simulink model "gm_Encoder_Zynq_V24"  (R2018a)
settings: Solver=ode3  StartTime=0.0  StopTime=SimulationsDauer  RelTol=1e-3  EnableMultiTasking=on
undefined symbols (not defined in the file or in its folder): DiscIntNeverNeededParam, f_ISR, IncPerTurn, n_max, OmegaPerOverSampl, OverSamplingFactor, OverSamplingFactorInverse, Periode, Phase_Delay_A, Phase_Delay_B, PolePair, QuadratureFactor, T_50MHz, T_mech, TestDrehzahl_rpm
libraries: simulink x2, dspswit3 x2, powerlib_meascontrol x2, simulink_extras x1, powerlib x1
(part 2 of 4)

== system gm_Encoder_Zynq_V24/IncreEncoder_V16/Check_Direction ==
  A : Inport
  B : Inport  Port=2
  Add : Sum  Inputs=+-  AccumDataTypeStr=fixdt(1,4,0)  OutDataTypeStr=fixdt(1,4,0)
  Add1 : Sum  Inputs=+-  AccumDataTypeStr=fixdt(1,4,0)  OutDataTypeStr=fixdt(1,4,0)
  Add2 : Sum  AccumDataTypeStr=fixdt(1,4,0)  OutDataTypeStr=fixdt(1,4,0)
  Change : Sum  AccumDataTypeStr=fixdt(1,4,0)  OutDataTypeStr=fixdt(1,4,0)
  Change1 : Delay  DelayLength=1
  Save_Direction : Switch  Criteria=u2 ~= 0  Threshold=0.1  OutDataTypeStr=Inherit: Inherit via back propagation
  Scope6 : Scope  NumInputPorts=4
  T_count_switch : Switch  Threshold=1  OutDataTypeStr=Inherit: Inherit via back propagation
  TrnLeft : Sum  Inputs=+-  AccumDataTypeStr=fixdt(1,4,0)  OutDataTypeStr=fixdt(1,4,0)
  TrnRight : Sum  Inputs=+-  AccumDataTypeStr=fixdt(1,4,0)  OutDataTypeStr=fixdt(1,4,0)
  TurnLeft : Constant  Value=-1  OutDataTypeStr=fixdt(1,4,0)  SampleTime=-1
  TurnRight : Constant  OutDataTypeStr=fixdt(1,4,0)  SampleTime=-1
  count_old : Delay  DelayLength=1
  count_old1 : Delay  DelayLength=1
  count_old2 : Delay  DelayLength=1
  count_old_switch : Switch  Criteria=u2 ~= 0  OutDataTypeStr=Inherit: Inherit via back propagation
  count_old_switch1 : Switch  Criteria=u2 ~= 0  OutDataTypeStr=Inherit: Inherit via back propagation
  new_value : Delay  DelayLength=1
  nothing : Constant  Value=0  OutDataTypeStr=fixdt(1,4,0)  SampleTime=-1
  nothing1 : Constant  Value=0  OutDataTypeStr=fixdt(1,4,0)  SampleTime=-1
  speed_old_switch : Switch  Threshold=1  OutDataTypeStr=Inherit: Inherit via back propagation
  Dir : Outport
  wires:
  count_old2/1 -> Dir/1, Save_Direction/3
  Change1/1 -> Save_Direction/2, Scope6/3
  Change/1 -> Change1/1
  Add2/1 -> new_value/1, Scope6/4
  speed_old_switch/1 -> Add2/2, Change/2
  nothing1/1 -> T_count_switch/3
  nothing/1 -> speed_old_switch/3
  TurnLeft/1 -> speed_old_switch/1
  TrnLeft/1 -> Scope6/2, speed_old_switch/2
  new_value/1 -> Save_Direction/1
  TrnRight/1 -> T_count_switch/2, Scope6/1
  Add1/1 -> count_old_switch1/2, TrnLeft/1
  count_old1/1 -> Add1/2, count_old_switch1/3
  count_old_switch1/1 -> count_old1/1
  B/1 -> count_old_switch1/1, Add1/1, TrnRight/2
  Save_Direction/1 -> count_old2/1
  T_count_switch/1 -> Add2/1, Change/1
  Add/1 -> count_old_switch/2, TrnRight/1
  TurnRight/1 -> T_count_switch/1
  count_old/1 -> Add/2, count_old_switch/3
  count_old_switch/1 -> count_old/1
  A/1 -> count_old_switch/1, Add/1, TrnLeft/2

== system gm_Encoder_Zynq_V24/IncreEncoder_V16/Counter_speed ==
  note: Count
  note: Reset
  note: Check if count is to big
  note: Check if count is to small
  note: 1 for one cycle if edge recognized
  Enable_ctr : Inport
  Reset : Inport  Port=2
  IncsPerTurn : Inport  Port=3
  Add1 : Sum  AccumDataTypeStr=int16  OutDataTypeStr=uint16
  Constant1 : Constant  Value=0  OutDataTypeStr=uint16  SampleTime=-1
  Constant2 : Constant  OutDataTypeStr=int8  SampleTime=-1
  Constant3 : Constant  Value=0  OutDataTypeStr=int8  SampleTime=-1
  Constant4 : Constant  Value=10  OutDataTypeStr=uint16  SampleTime=-1
  Detec_edge : Sum  Inputs=+-  AccumDataTypeStr=int8  OutDataTypeStr=int8
  Relational Operator : RelationalOperator  OutDataTypeStr=boolean  RndMeth=Nearest
  Reset_flag : Sum  Inputs=+-  AccumDataTypeStr=uint8  OutDataTypeStr=uint8
  Reset_when_overflow : Sum
  Resett_switch1 : Switch  Criteria=u2 ~= 0
  Resett_switch2 : Switch  Criteria=u2 ~= 0
  reset_old{,1..3} (4 alike) : Delay  DelayLength=1
  reset_old_switch : Switch  Criteria=u2 ~= 0
  reset_old_switch1 : Switch  Criteria=u2 ~= 0
  speed_old_switch1 : Switch  Threshold=1
  count : Outport
  wires:
  reset_old3/1 -> Relational Operator/2
  Resett_switch2/1 -> Resett_switch1/3
  IncsPerTurn/1 -> Reset_when_overflow/2
  Constant1/1 -> Resett_switch1/1, Resett_switch2/1
  Relational Operator/1 -> Resett_switch1/2
  Resett_switch1/1 -> reset_old2/1
  Reset_when_overflow/1 -> reset_old3/1
  Constant4/1 -> Reset_when_overflow/1
  Constant2/1 -> speed_old_switch1/1
  Constant3/1 -> speed_old_switch1/3
  speed_old_switch1/1 -> Add1/1
  reset_old2/1 -> count/1, Add1/2, Relational Operator/1
  Add1/1 -> Resett_switch2/3
  Detec_edge/1 -> reset_old_switch1/2, speed_old_switch1/2  "1 for one cycle if edge recognized"
  reset_old1/1 -> Detec_edge/2, reset_old_switch1/3
  reset_old_switch1/1 -> reset_old1/1
  Enable_ctr/1 -> reset_old_switch1/1, Detec_edge/1
  Reset_flag/1 -> Resett_switch2/2, reset_old_switch/2
  reset_old/1 -> Reset_flag/2, reset_old_switch/3
  reset_old_switch/1 -> reset_old/1
  Reset/1 -> reset_old_switch/1, Reset_flag/1

== system gm_Encoder_Zynq_V24/IncreEncoder_V16/Counter_theta ==
  note: Check if count is to small
  note: Check if count is to big
  note: Count
  note: Reset
  note: 1 for one cycle if edge recognized
  Enable_ctr : Inport
  Reset : Inport  Port=2
  IncsPerTurn : Inport  Port=3
  Dir : Inport  Port=4
  Add1 : Sum  AccumDataTypeStr=int16  OutDataTypeStr=int16
  Constant1 : Constant  Value=0  OutDataTypeStr=int16  SampleTime=-1
  Constant2 : Constant  OutDataTypeStr=int16  SampleTime=-1
  Constant3 : Constant  Value=0  OutDataTypeStr=int16  SampleTime=-1
  Constant4 : Constant  Value=10  OutDataTypeStr=int16  SampleTime=-1
  Constant5 : Constant  Value=-1  OutDataTypeStr=int16  SampleTime=-1
  Detec_edge : Sum  Inputs=+-  AccumDataTypeStr=int8  OutDataTypeStr=int8
  Relational Operator : RelationalOperator  Operator=>  OutDataTypeStr=boolean  RndMeth=Nearest
  Relational Operator1 : RelationalOperator  Operator=<=  OutDataTypeStr=boolean  RndMeth=Nearest
  Reset_flag : Sum  Inputs=+-  AccumDataTypeStr=uint8  OutDataTypeStr=uint8
  Reset_when_overflow : Sum  OutDataTypeStr=int16
  Resett_switch1 : Switch  Criteria=u2 ~= 0  OutDataTypeStr=int16
  Resett_switch2 : Switch  Criteria=u2 ~= 0  OutDataTypeStr=int16
  Resett_switch3 : Switch  Criteria=u2 ~= 0  OutDataTypeStr=int16
  only_use_for_neg_speed : Switch  Threshold=1
  reset_old{,1..6} (7 alike) : Delay  DelayLength=1
  reset_old_switch : Switch  Criteria=u2 ~= 0
  reset_old_switch1 : Switch  Criteria=u2 ~= 0
  speed_old_switch1 : Switch  Criteria=u2 ~= 0
  speed_old_switch2 : Switch  Threshold=1
  count : Outport
  wires:
  reset_old6/1 -> speed_old_switch2/2, only_use_for_neg_speed/2
  reset_old5/1 -> Relational Operator/2
  reset_old4/1 -> speed_old_switch1/1
  only_use_for_neg_speed/1 -> Resett_switch3/2
  Relational Operator1/1 -> only_use_for_neg_speed/3
  reset_old2/1 -> Relational Operator1/1
  Resett_switch2/1 -> Resett_switch3/3
  Resett_switch3/1 -> Resett_switch1/3, reset_old2/1
  Constant1/1 -> Relational Operator1/2, only_use_for_neg_speed/1, Resett_switch1/1, Resett_switch2/1
  Relational Operator/1 -> Resett_switch1/2
  Resett_switch1/1 -> reset_old3/1
  reset_old3/1 -> Relational Operator/1, count/1, Add1/2
  speed_old_switch2/1 -> reset_old4/1
  Constant5/1 -> speed_old_switch2/3
  Dir/1 -> reset_old6/1
  IncsPerTurn/1 -> Reset_when_overflow/2, Resett_switch3/1
  Reset_when_overflow/1 -> reset_old5/1
  Constant4/1 -> Reset_when_overflow/1
  Constant2/1 -> speed_old_switch2/1
  Constant3/1 -> speed_old_switch1/3
  speed_old_switch1/1 -> Add1/1
  Add1/1 -> Resett_switch2/3
  Detec_edge/1 -> reset_old_switch1/2, speed_old_switch1/2  "1 for one cycle if edge recognized"
  reset_old1/1 -> Detec_edge/2, reset_old_switch1/3
  reset_old_switch1/1 -> reset_old1/1
  Enable_ctr/1 -> reset_old_switch1/1, Detec_edge/1
  Reset_flag/1 -> Resett_switch2/2, reset_old_switch/2
  reset_old/1 -> Reset_flag/2, reset_old_switch/3
  reset_old_switch/1 -> reset_old/1
  Reset/1 -> reset_old_switch/1, Reset_flag/1

== system gm_Encoder_Zynq_V24/IncreEncoder_V16/Counter_theta_ele ==
  note: Check if count is to small
  note: Check if count is to big
  note: Count
  note: Reset
  note: 1 for one cycle if edge recognized
  Enable_ctr : Inport
  Reset : Inport  Port=2
  IncsPerTurn : Inport  Port=3
  Dir : Inport  Port=4
  Add1 : Sum  AccumDataTypeStr=int16  OutDataTypeStr=int16
  Constant1 : Constant  Value=0  OutDataTypeStr=int16  SampleTime=-1
  Constant2 : Constant  OutDataTypeStr=int16  SampleTime=-1
  Constant3 : Constant  Value=0  OutDataTypeStr=int16  SampleTime=-1
  Constant5 : Constant  Value=-1  OutDataTypeStr=int16  SampleTime=-1
  Detec_edge : Sum  Inputs=+-  AccumDataTypeStr=int8  OutDataTypeStr=int8
  Relational Operator : RelationalOperator  Operator=>  OutDataTypeStr=boolean  RndMeth=Nearest
  Relational Operator1 : RelationalOperator  Operator=<=  OutDataTypeStr=boolean  RndMeth=Nearest
  Reset_flag : Sum  Inputs=+-  AccumDataTypeStr=uint8  OutDataTypeStr=uint8
  Resett_switch1 : Switch  Criteria=u2 ~= 0  OutDataTypeStr=int16
  Resett_switch2 : Switch  Criteria=u2 ~= 0  OutDataTypeStr=int16
  Resett_switch3 : Switch  Criteria=u2 ~= 0  OutDataTypeStr=int16
  only_use_for_neg_speed : Switch  Threshold=1
  reset_old{,1..5} (6 alike) : Delay  DelayLength=1
  reset_old_switch : Switch  Criteria=u2 ~= 0
  reset_old_switch1 : Switch  Criteria=u2 ~= 0
  speed_old_switch1 : Switch  Criteria=u2 ~= 0
  speed_old_switch2 : Switch  Threshold=1
  count : Outport
  wires:
  reset_old5/1 -> only_use_for_neg_speed/2, speed_old_switch2/2
  reset_old4/1 -> speed_old_switch1/1
  only_use_for_neg_speed/1 -> Resett_switch3/2
  Relational Operator1/1 -> only_use_for_neg_speed/3
  reset_old2/1 -> Relational Operator1/1
  Resett_switch2/1 -> Resett_switch3/3
  Resett_switch3/1 -> Resett_switch1/3, reset_old2/1
  Constant1/1 -> Resett_switch1/1, Relational Operator1/2, only_use_for_neg_speed/1, Resett_switch2/1
  Relational Operator/1 -> Resett_switch1/2
  Resett_switch1/1 -> reset_old3/1
  reset_old3/1 -> Relational Operator/1, count/1, Add1/2
  speed_old_switch2/1 -> reset_old4/1
  Constant5/1 -> speed_old_switch2/3
  Dir/1 -> reset_old5/1
  IncsPerTurn/1 -> Relational Operator/2, Resett_switch3/1
  Constant2/1 -> speed_old_switch2/1
  Constant3/1 -> speed_old_switch1/3
  speed_old_switch1/1 -> Add1/1
  Add1/1 -> Resett_switch2/3
  Detec_edge/1 -> reset_old_switch1/2, speed_old_switch1/2  "1 for one cycle if edge recognized"
  reset_old1/1 -> Detec_edge/2, reset_old_switch1/3
  reset_old_switch1/1 -> reset_old1/1
  Enable_ctr/1 -> reset_old_switch1/1, Detec_edge/1
  Reset_flag/1 -> Resett_switch2/2, reset_old_switch/2
  reset_old/1 -> Reset_flag/2, reset_old_switch/3
  reset_old_switch/1 -> reset_old/1
  Reset/1 -> reset_old_switch/1, Reset_flag/1

== system gm_Encoder_Zynq_V24/IncreEncoder_V16/n_aus_theta ==
  count : Inport
  IncsPerTurn : Inport  Port=2
  T : Inport  Port=3
  Add : Sum  Inputs=+-
  Add1 : Sum
  Constant : Constant  Value=0  OutDataTypeStr=fixdt(0,30,24)  SampleTime=-1
  Constant1 : Constant  Value=0  OutDataTypeStr=fixdt(0,30,24)  SampleTime=-1
  Constant2 : Constant  Value=0  OutDataTypeStr=fixdt(0,30,24)  SampleTime=-1
  Gain : Gain  Gain=0.001  ParamDataTypeStr=fixdt(0,16)  OutMin=0  OutMax=0.001*2^16  OutDataTypeStr=fixdt(0,18)
  Product : Product  OutDataTypeStr=Inherit: Same as first input
  ProtectOverflow_T_count : Switch  Threshold=50
  ProtectOverflow_rps : Switch  Threshold=50  OutDataTypeStr=fixdt(0,30,24)
  T_count : Delay  DelayLength=1
  T_count_switch : Switch  Criteria=u2 ~= 0
  count_old : Delay  DelayLength=1
  count_old_switch : Switch  Criteria=u2 ~= 0
  speed_old : Delay  DelayLength=1
  speed_old_switch : Switch  Criteria=u2 ~= 0
  rps : Outport
  wires:
  T_count_switch/1 -> ProtectOverflow_T_count/3, ProtectOverflow_T_count/2, ProtectOverflow_rps/2
  count/1 -> count_old_switch/1, Add/1
  Add1/1 -> T_count_switch/3, Product/1
  Product/1 -> speed_old_switch/1
  T_count/1 -> Add1/2
  ProtectOverflow_T_count/1 -> T_count/1
  T/1 -> Add1/1
  Gain/1 -> Product/2
  IncsPerTurn/1 -> Gain/1
  speed_old/1 -> speed_old_switch/3
  speed_old_switch/1 -> speed_old/1, ProtectOverflow_rps/3
  Constant2/1 -> ProtectOverflow_rps/1
  ProtectOverflow_rps/1 -> rps/1
  Constant1/1 -> ProtectOverflow_T_count/1
  Add/1 -> T_count_switch/2, count_old_switch/2, speed_old_switch/2
  Constant/1 -> T_count_switch/1
  count_old/1 -> Add/2, count_old_switch/3
  count_old_switch/1 -> count_old/1

== system gm_Encoder_Zynq_V24/IncreEncoder_V18/Check_Direction ==
  A : Inport
  B : Inport  Port=2
  Add : Sum  Inputs=+-  AccumDataTypeStr=fixdt(1,4,0)  OutDataTypeStr=fixdt(1,4,0)
  Add1 : Sum  Inputs=+-  AccumDataTypeStr=fixdt(1,4,0)  OutDataTypeStr=fixdt(1,4,0)
  Add2 : Sum  AccumDataTypeStr=fixdt(1,4,0)  OutDataTypeStr=fixdt(1,4,0)
  Change : Sum  AccumDataTypeStr=fixdt(1,4,0)  OutDataTypeStr=fixdt(1,4,0)
  Change1 : Delay  DelayLength=1
  Save_Direction : Switch  Criteria=u2 ~= 0  Threshold=0.1  OutDataTypeStr=Inherit: Inherit via back propagation
  Scope6 : Scope  NumInputPorts=4
  T_count_switch : Switch  Threshold=1  OutDataTypeStr=Inherit: Inherit via back propagation
  TrnLeft : Sum  Inputs=+-  AccumDataTypeStr=fixdt(1,4,0)  OutDataTypeStr=fixdt(1,4,0)
  TrnRight : Sum  Inputs=+-  AccumDataTypeStr=fixdt(1,4,0)  OutDataTypeStr=fixdt(1,4,0)
  TurnLeft : Constant  Value=-1  OutDataTypeStr=fixdt(1,4,0)  SampleTime=-1
  TurnRight : Constant  OutDataTypeStr=fixdt(1,4,0)  SampleTime=-1
  count_old : Delay  DelayLength=1
  count_old1 : Delay  DelayLength=1
  count_old2 : Delay  DelayLength=1
  count_old_switch : Switch  Criteria=u2 ~= 0  OutDataTypeStr=Inherit: Inherit via back propagation
  count_old_switch1 : Switch  Criteria=u2 ~= 0  OutDataTypeStr=Inherit: Inherit via back propagation
  new_value : Delay  DelayLength=1
  nothing : Constant  Value=0  OutDataTypeStr=fixdt(1,4,0)  SampleTime=-1
  nothing1 : Constant  Value=0  OutDataTypeStr=fixdt(1,4,0)  SampleTime=-1
  speed_old_switch : Switch  Threshold=1  OutDataTypeStr=Inherit: Inherit via back propagation
  Dir : Outport
  wires:
  count_old2/1 -> Dir/1, Save_Direction/3
  Change1/1 -> Save_Direction/2, Scope6/3
  Change/1 -> Change1/1
  Add2/1 -> new_value/1, Scope6/4
  speed_old_switch/1 -> Add2/2, Change/2
  nothing1/1 -> T_count_switch/3
  nothing/1 -> speed_old_switch/3
  TurnLeft/1 -> speed_old_switch/1
  TrnLeft/1 -> Scope6/2, speed_old_switch/2
  new_value/1 -> Save_Direction/1
  TrnRight/1 -> T_count_switch/2, Scope6/1
  Add1/1 -> count_old_switch1/2, TrnLeft/1
  count_old1/1 -> Add1/2, count_old_switch1/3
  count_old_switch1/1 -> count_old1/1
  B/1 -> count_old_switch1/1, Add1/1, TrnRight/2
  Save_Direction/1 -> count_old2/1
  T_count_switch/1 -> Add2/1, Change/1
  Add/1 -> count_old_switch/2, TrnRight/1
  TurnRight/1 -> T_count_switch/1
  count_old/1 -> Add/2, count_old_switch/3
  count_old_switch/1 -> count_old/1
  A/1 -> count_old_switch/1, Add/1, TrnLeft/2

== system gm_Encoder_Zynq_V24/IncreEncoder_V18/Counter_speed ==
  note: Count
  note: Reset
  note: Check if count is to big
  note: Check if count is to small
  note: 1 for one cycle if edge recognized
  Enable_ctr : Inport
  Reset : Inport  Port=2
  IncsPerTurn : Inport  Port=3
  Add1 : Sum  AccumDataTypeStr=int16  OutDataTypeStr=uint16
  Constant1 : Constant  Value=0  OutDataTypeStr=uint16  SampleTime=-1
  Constant2 : Constant  OutDataTypeStr=int8  SampleTime=-1
  Constant3 : Constant  Value=0  OutDataTypeStr=int8  SampleTime=-1
  Constant4 : Constant  Value=10  OutDataTypeStr=uint16  SampleTime=-1
  Detec_edge : Sum  Inputs=+-  AccumDataTypeStr=int8  OutDataTypeStr=int8
  Relational Operator : RelationalOperator  OutDataTypeStr=boolean  RndMeth=Nearest
  Reset_flag : Sum  Inputs=+-  AccumDataTypeStr=uint8  OutDataTypeStr=uint8
  Reset_when_overflow : Sum
  Resett_switch1 : Switch  Criteria=u2 ~= 0
  Resett_switch2 : Switch  Criteria=u2 ~= 0
  reset_old{,1..3} (4 alike) : Delay  DelayLength=1
  reset_old_switch : Switch  Criteria=u2 ~= 0
  reset_old_switch1 : Switch  Criteria=u2 ~= 0
  speed_old_switch1 : Switch  Threshold=1
  count : Outport
  wires:
  reset_old3/1 -> Relational Operator/2
  Resett_switch2/1 -> Resett_switch1/3
  IncsPerTurn/1 -> Reset_when_overflow/2
  Constant1/1 -> Resett_switch1/1, Resett_switch2/1
  Relational Operator/1 -> Resett_switch1/2
  Resett_switch1/1 -> reset_old2/1
  Reset_when_overflow/1 -> reset_old3/1
  Constant4/1 -> Reset_when_overflow/1
  Constant2/1 -> speed_old_switch1/1
  Constant3/1 -> speed_old_switch1/3
  speed_old_switch1/1 -> Add1/1
  reset_old2/1 -> count/1, Add1/2, Relational Operator/1
  Add1/1 -> Resett_switch2/3
  Detec_edge/1 -> reset_old_switch1/2, speed_old_switch1/2  "1 for one cycle if edge recognized"
  reset_old1/1 -> Detec_edge/2, reset_old_switch1/3
  reset_old_switch1/1 -> reset_old1/1
  Enable_ctr/1 -> reset_old_switch1/1, Detec_edge/1
  Reset_flag/1 -> Resett_switch2/2, reset_old_switch/2
  reset_old/1 -> Reset_flag/2, reset_old_switch/3
  reset_old_switch/1 -> reset_old/1
  Reset/1 -> reset_old_switch/1, Reset_flag/1

== system gm_Encoder_Zynq_V24/IncreEncoder_V18/Counter_theta ==
  note: Check if count is to small
  note: Check if count is to big
  note: Count
  note: Reset
  note: 1 for one cycle if edge recognized
  Enable_ctr : Inport
  Reset : Inport  Port=2
  IncsPerTurn : Inport  Port=3
  Dir : Inport  Port=4
  Add1 : Sum  AccumDataTypeStr=int16  OutDataTypeStr=int16
  Constant1 : Constant  Value=0  OutDataTypeStr=int16  SampleTime=-1
  Constant2 : Constant  OutDataTypeStr=int16  SampleTime=-1
  Constant3 : Constant  Value=0  OutDataTypeStr=int16  SampleTime=-1
  Constant4 : Constant  Value=10  OutDataTypeStr=int16  SampleTime=-1
  Constant5 : Constant  Value=-1  OutDataTypeStr=int16  SampleTime=-1
  Detec_edge : Sum  Inputs=+-  AccumDataTypeStr=int8  OutDataTypeStr=int8
  Relational Operator : RelationalOperator  Operator=>  OutDataTypeStr=boolean  RndMeth=Nearest
  Relational Operator1 : RelationalOperator  Operator=<=  OutDataTypeStr=boolean  RndMeth=Nearest
  Reset_flag : Sum  Inputs=+-  AccumDataTypeStr=uint8  OutDataTypeStr=uint8
  Reset_when_overflow : Sum  OutDataTypeStr=int16
  Resett_switch1 : Switch  Criteria=u2 ~= 0  OutDataTypeStr=int16
  Resett_switch2 : Switch  Criteria=u2 ~= 0  OutDataTypeStr=int16
  Resett_switch3 : Switch  Criteria=u2 ~= 0  OutDataTypeStr=int16
  only_use_for_neg_speed : Switch  Threshold=1
  reset_old{,1..6} (7 alike) : Delay  DelayLength=1
  reset_old_switch : Switch  Criteria=u2 ~= 0
  reset_old_switch1 : Switch  Criteria=u2 ~= 0
  speed_old_switch1 : Switch  Criteria=u2 ~= 0
  speed_old_switch2 : Switch  Threshold=1
  count : Outport
  wires:
  reset_old6/1 -> speed_old_switch2/2, only_use_for_neg_speed/2
  reset_old5/1 -> Relational Operator/2
  reset_old4/1 -> speed_old_switch1/1
  only_use_for_neg_speed/1 -> Resett_switch3/2
  Relational Operator1/1 -> only_use_for_neg_speed/3
  reset_old2/1 -> Relational Operator1/1
  Resett_switch2/1 -> Resett_switch3/3
  Resett_switch3/1 -> Resett_switch1/3, reset_old2/1
  Constant1/1 -> Relational Operator1/2, only_use_for_neg_speed/1, Resett_switch1/1, Resett_switch2/1
  Relational Operator/1 -> Resett_switch1/2
  Resett_switch1/1 -> reset_old3/1
  reset_old3/1 -> Relational Operator/1, count/1, Add1/2
  speed_old_switch2/1 -> reset_old4/1
  Constant5/1 -> speed_old_switch2/3
  Dir/1 -> reset_old6/1
  IncsPerTurn/1 -> Reset_when_overflow/2, Resett_switch3/1
  Reset_when_overflow/1 -> reset_old5/1
  Constant4/1 -> Reset_when_overflow/1
  Constant2/1 -> speed_old_switch2/1
  Constant3/1 -> speed_old_switch1/3
  speed_old_switch1/1 -> Add1/1
  Add1/1 -> Resett_switch2/3
  Detec_edge/1 -> reset_old_switch1/2, speed_old_switch1/2  "1 for one cycle if edge recognized"
  reset_old1/1 -> Detec_edge/2, reset_old_switch1/3
  reset_old_switch1/1 -> reset_old1/1
  Enable_ctr/1 -> reset_old_switch1/1, Detec_edge/1
  Reset_flag/1 -> Resett_switch2/2, reset_old_switch/2
  reset_old/1 -> Reset_flag/2, reset_old_switch/3
  reset_old_switch/1 -> reset_old/1
  Reset/1 -> reset_old_switch/1, Reset_flag/1

== system gm_Encoder_Zynq_V24/IncreEncoder_V18/Counter_theta_ele ==
  note: Check if count is to small
  note: Check if count is to big
  note: Count
  note: Reset
  note: 1 for one cycle if edge recognized
  Enable_ctr : Inport
  Reset : Inport  Port=2
  IncsPerTurn : Inport  Port=3
  Dir : Inport  Port=4
  Add1 : Sum  AccumDataTypeStr=int16  OutDataTypeStr=int16
  Constant1 : Constant  Value=0  OutDataTypeStr=int16  SampleTime=-1
  Constant2 : Constant  OutDataTypeStr=int16  SampleTime=-1
  Constant3 : Constant  Value=0  OutDataTypeStr=int16  SampleTime=-1
  Constant5 : Constant  Value=-1  OutDataTypeStr=int16  SampleTime=-1
  Detec_edge : Sum  Inputs=+-  AccumDataTypeStr=int8  OutDataTypeStr=int8
  Relational Operator : RelationalOperator  Operator=>  OutDataTypeStr=boolean  RndMeth=Nearest
  Relational Operator1 : RelationalOperator  Operator=<=  OutDataTypeStr=boolean  RndMeth=Nearest
  Reset_flag : Sum  Inputs=+-  AccumDataTypeStr=uint8  OutDataTypeStr=uint8
  Resett_switch1 : Switch  Criteria=u2 ~= 0  OutDataTypeStr=int16
  Resett_switch2 : Switch  Criteria=u2 ~= 0  OutDataTypeStr=int16
  Resett_switch3 : Switch  Criteria=u2 ~= 0  OutDataTypeStr=int16
  only_use_for_neg_speed : Switch  Threshold=1
  reset_old{,1..5} (6 alike) : Delay  DelayLength=1
  reset_old_switch : Switch  Criteria=u2 ~= 0
  reset_old_switch1 : Switch  Criteria=u2 ~= 0
  speed_old_switch1 : Switch  Criteria=u2 ~= 0
  speed_old_switch2 : Switch  Threshold=1
  count : Outport
  wires:
  reset_old5/1 -> only_use_for_neg_speed/2, speed_old_switch2/2
  reset_old4/1 -> speed_old_switch1/1
  only_use_for_neg_speed/1 -> Resett_switch3/2
  Relational Operator1/1 -> only_use_for_neg_speed/3
  reset_old2/1 -> Relational Operator1/1
  Resett_switch2/1 -> Resett_switch3/3
  Resett_switch3/1 -> Resett_switch1/3, reset_old2/1
  Constant1/1 -> Resett_switch1/1, Relational Operator1/2, only_use_for_neg_speed/1, Resett_switch2/1
  Relational Operator/1 -> Resett_switch1/2
  Resett_switch1/1 -> reset_old3/1
  reset_old3/1 -> Relational Operator/1, count/1, Add1/2
  speed_old_switch2/1 -> reset_old4/1
  Constant5/1 -> speed_old_switch2/3
  Dir/1 -> reset_old5/1
  IncsPerTurn/1 -> Relational Operator/2, Resett_switch3/1
  Constant2/1 -> speed_old_switch2/1
  Constant3/1 -> speed_old_switch1/3
  speed_old_switch1/1 -> Add1/1
  Add1/1 -> Resett_switch2/3
  Detec_edge/1 -> reset_old_switch1/2, speed_old_switch1/2  "1 for one cycle if edge recognized"
  reset_old1/1 -> Detec_edge/2, reset_old_switch1/3
  reset_old_switch1/1 -> reset_old1/1
  Enable_ctr/1 -> reset_old_switch1/1, Detec_edge/1
  Reset_flag/1 -> Resett_switch2/2, reset_old_switch/2
  reset_old/1 -> Reset_flag/2, reset_old_switch/3
  reset_old_switch/1 -> reset_old/1
  Reset/1 -> reset_old_switch/1, Reset_flag/1

== system gm_Encoder_Zynq_V24/IncreEncoder_V18/n_aus_theta ==
  count : Inport
  IncsPerTurn : Inport  Port=2
  T : Inport  Port=3
  Add : Sum  Inputs=+-
  Add1 : Sum
  Constant : Constant  Value=0  OutDataTypeStr=fixdt(0,30,24)  SampleTime=-1
  Constant1 : Constant  Value=0  OutDataTypeStr=fixdt(0,30,24)  SampleTime=-1
  Constant2 : Constant  Value=0  OutDataTypeStr=fixdt(0,30,24)  SampleTime=-1
  Gain : Gain  Gain=0.001  ParamDataTypeStr=fixdt(0,16)  OutMin=0  OutMax=0.001*2^16  OutDataTypeStr=fixdt(0,18)
  Product : Product  OutDataTypeStr=Inherit: Same as first input
  ProtectOverflow_T_count : Switch  Threshold=50
  ProtectOverflow_rps : Switch  Threshold=50  OutDataTypeStr=fixdt(0,30,24)
  T_count : Delay  DelayLength=1
  T_count_switch : Switch  Criteria=u2 ~= 0
  count_old : Delay  DelayLength=1
  count_old_switch : Switch  Criteria=u2 ~= 0
  speed_old : Delay  DelayLength=1
  speed_old_switch : Switch  Criteria=u2 ~= 0
  rps : Outport
  wires:
  T_count_switch/1 -> ProtectOverflow_T_count/3, ProtectOverflow_T_count/2, ProtectOverflow_rps/2
  count/1 -> count_old_switch/1, Add/1
  Add1/1 -> T_count_switch/3, Product/1
  Product/1 -> speed_old_switch/1
  T_count/1 -> Add1/2
  ProtectOverflow_T_count/1 -> T_count/1
  T/1 -> Add1/1
  Gain/1 -> Product/2
  IncsPerTurn/1 -> Gain/1
  speed_old/1 -> speed_old_switch/3
  speed_old_switch/1 -> speed_old/1, ProtectOverflow_rps/3
  Constant2/1 -> ProtectOverflow_rps/1
  ProtectOverflow_rps/1 -> rps/1
  Constant1/1 -> ProtectOverflow_T_count/1
  Add/1 -> T_count_switch/2, count_old_switch/2, speed_old_switch/2
  Constant/1 -> T_count_switch/1
  count_old/1 -> Add/2, count_old_switch/3
  count_old_switch/1 -> count_old/1

== system gm_Encoder_Zynq_V24/IncreEncoder_V19/Check_Direction ==
  A : Inport
  B : Inport  Port=2
  Add : Sum  Inputs=+-  AccumDataTypeStr=fixdt(1,4,0)  OutDataTypeStr=fixdt(1,4,0)
  Add1 : Sum  Inputs=+-  AccumDataTypeStr=fixdt(1,4,0)  OutDataTypeStr=fixdt(1,4,0)
  Add2 : Sum  AccumDataTypeStr=fixdt(1,4,0)  OutDataTypeStr=fixdt(1,4,0)
  Change : Sum  AccumDataTypeStr=fixdt(1,4,0)  OutDataTypeStr=fixdt(1,4,0)
  Change1 : Delay  DelayLength=1
  Save_Direction : Switch  Criteria=u2 ~= 0  Threshold=0.1  OutDataTypeStr=Inherit: Inherit via back propagation
  Scope6 : Scope  NumInputPorts=4
  T_count_switch : Switch  Threshold=1  OutDataTypeStr=Inherit: Inherit via back propagation
  TrnLeft : Sum  Inputs=+-  AccumDataTypeStr=fixdt(1,4,0)  OutDataTypeStr=fixdt(1,4,0)
  TrnRight : Sum  Inputs=+-  AccumDataTypeStr=fixdt(1,4,0)  OutDataTypeStr=fixdt(1,4,0)
  TurnLeft : Constant  Value=-1  OutDataTypeStr=fixdt(1,4,0)  SampleTime=-1
  TurnRight : Constant  OutDataTypeStr=fixdt(1,4,0)  SampleTime=-1
  count_old : Delay  DelayLength=1
  count_old1 : Delay  DelayLength=1
  count_old2 : Delay  DelayLength=1
  count_old_switch : Switch  Criteria=u2 ~= 0  OutDataTypeStr=Inherit: Inherit via back propagation
  count_old_switch1 : Switch  Criteria=u2 ~= 0  OutDataTypeStr=Inherit: Inherit via back propagation
  new_value : Delay  DelayLength=1
  nothing : Constant  Value=0  OutDataTypeStr=fixdt(1,4,0)  SampleTime=-1
  nothing1 : Constant  Value=0  OutDataTypeStr=fixdt(1,4,0)  SampleTime=-1
  speed_old_switch : Switch  Threshold=1  OutDataTypeStr=Inherit: Inherit via back propagation
  Dir : Outport
  wires:
  count_old2/1 -> Dir/1, Save_Direction/3
  Change1/1 -> Save_Direction/2, Scope6/3
  Change/1 -> Change1/1
  Add2/1 -> new_value/1, Scope6/4
  speed_old_switch/1 -> Add2/2, Change/2
  nothing1/1 -> T_count_switch/3
  nothing/1 -> speed_old_switch/3
  TurnLeft/1 -> speed_old_switch/1
  TrnLeft/1 -> Scope6/2, speed_old_switch/2
  new_value/1 -> Save_Direction/1
  TrnRight/1 -> T_count_switch/2, Scope6/1
  Add1/1 -> count_old_switch1/2, TrnLeft/1
  count_old1/1 -> Add1/2, count_old_switch1/3
  count_old_switch1/1 -> count_old1/1
  B/1 -> count_old_switch1/1, Add1/1, TrnRight/2
  Save_Direction/1 -> count_old2/1
  T_count_switch/1 -> Add2/1, Change/1
  Add/1 -> count_old_switch/2, TrnRight/1
  TurnRight/1 -> T_count_switch/1
  count_old/1 -> Add/2, count_old_switch/3
  count_old_switch/1 -> count_old/1
  A/1 -> count_old_switch/1, Add/1, TrnLeft/2

== system gm_Encoder_Zynq_V24/IncreEncoder_V19/Counter_speed ==
  note: Count
  note: Reset
  note: Check if count is to big
  note: Check if count is to small
  note: 1 for one cycle if edge recognized
  Enable_ctr : Inport
  Reset : Inport  Port=2
  IncsPerTurn : Inport  Port=3
  Add1 : Sum  AccumDataTypeStr=int16  OutDataTypeStr=uint16
  Constant1 : Constant  Value=0  OutDataTypeStr=uint16  SampleTime=-1
  Constant2 : Constant  OutDataTypeStr=int8  SampleTime=-1
  Constant3 : Constant  Value=0  OutDataTypeStr=int8  SampleTime=-1
  Constant4 : Constant  Value=10  OutDataTypeStr=uint16  SampleTime=-1
  Detec_edge : Sum  Inputs=+-  AccumDataTypeStr=int8  OutDataTypeStr=int8
  Relational Operator : RelationalOperator  OutDataTypeStr=boolean  RndMeth=Nearest
  Reset_flag : Sum  Inputs=+-  AccumDataTypeStr=uint8  OutDataTypeStr=uint8
  Reset_when_overflow : Sum
  Resett_switch1 : Switch  Criteria=u2 ~= 0
  Resett_switch2 : Switch  Criteria=u2 ~= 0
  reset_old{,1..3} (4 alike) : Delay  DelayLength=1
  reset_old_switch : Switch  Criteria=u2 ~= 0
  reset_old_switch1 : Switch  Criteria=u2 ~= 0
  speed_old_switch1 : Switch  Threshold=1
  count : Outport
  wires:
  reset_old3/1 -> Relational Operator/2
  Resett_switch2/1 -> Resett_switch1/3
  IncsPerTurn/1 -> Reset_when_overflow/2
  Constant1/1 -> Resett_switch1/1, Resett_switch2/1
  Relational Operator/1 -> Resett_switch1/2
  Resett_switch1/1 -> reset_old2/1
  Reset_when_overflow/1 -> reset_old3/1
  Constant4/1 -> Reset_when_overflow/1
  Constant2/1 -> speed_old_switch1/1
  Constant3/1 -> speed_old_switch1/3
  speed_old_switch1/1 -> Add1/1
  reset_old2/1 -> count/1, Add1/2, Relational Operator/1
  Add1/1 -> Resett_switch2/3
  Detec_edge/1 -> reset_old_switch1/2, speed_old_switch1/2  "1 for one cycle if edge recognized"
  reset_old1/1 -> Detec_edge/2, reset_old_switch1/3
  reset_old_switch1/1 -> reset_old1/1
  Enable_ctr/1 -> reset_old_switch1/1, Detec_edge/1
  Reset_flag/1 -> Resett_switch2/2, reset_old_switch/2
  reset_old/1 -> Reset_flag/2, reset_old_switch/3
  reset_old_switch/1 -> reset_old/1
  Reset/1 -> reset_old_switch/1, Reset_flag/1

== system gm_Encoder_Zynq_V24/IncreEncoder_V19/Counter_theta ==
  note: Check if count is to small
  note: Check if count is to big
  note: Count
  note: Reset
  note: 1 for one cycle if edge recognized
  Enable_ctr : Inport
  Reset : Inport  Port=2
  IncsPerTurn : Inport  Port=3
  Dir : Inport  Port=4
  Add1 : Sum  AccumDataTypeStr=int16  OutDataTypeStr=int16
  Constant1 : Constant  Value=0  OutDataTypeStr=int16  SampleTime=-1
  Constant2 : Constant  OutDataTypeStr=int16  SampleTime=-1
  Constant3 : Constant  Value=0  OutDataTypeStr=int16  SampleTime=-1
  Constant4 : Constant  Value=10  OutDataTypeStr=int16  SampleTime=-1
  Constant5 : Constant  Value=-1  OutDataTypeStr=int16  SampleTime=-1
  Detec_edge : Sum  Inputs=+-  AccumDataTypeStr=int8  OutDataTypeStr=int8
  Relational Operator : RelationalOperator  Operator=>  OutDataTypeStr=boolean  RndMeth=Nearest
  Relational Operator1 : RelationalOperator  Operator=<=  OutDataTypeStr=boolean  RndMeth=Nearest
  Reset_flag : Sum  Inputs=+-  AccumDataTypeStr=uint8  OutDataTypeStr=uint8
  Reset_when_overflow : Sum  OutDataTypeStr=int16
  Resett_switch1 : Switch  Criteria=u2 ~= 0  OutDataTypeStr=int16
  Resett_switch2 : Switch  Criteria=u2 ~= 0  OutDataTypeStr=int16
  Resett_switch3 : Switch  Criteria=u2 ~= 0  OutDataTypeStr=int16
  only_use_for_neg_speed : Switch  Threshold=1
  reset_old{,1..6} (7 alike) : Delay  DelayLength=1
  reset_old_switch : Switch  Criteria=u2 ~= 0
  reset_old_switch1 : Switch  Criteria=u2 ~= 0
  speed_old_switch1 : Switch  Criteria=u2 ~= 0
  speed_old_switch2 : Switch  Threshold=1
  count : Outport
  wires:
  reset_old6/1 -> speed_old_switch2/2, only_use_for_neg_speed/2
  reset_old5/1 -> Relational Operator/2
  reset_old4/1 -> speed_old_switch1/1
  only_use_for_neg_speed/1 -> Resett_switch3/2
  Relational Operator1/1 -> only_use_for_neg_speed/3
  reset_old2/1 -> Relational Operator1/1
  Resett_switch2/1 -> Resett_switch3/3
  Resett_switch3/1 -> Resett_switch1/3, reset_old2/1
  Constant1/1 -> Relational Operator1/2, only_use_for_neg_speed/1, Resett_switch1/1, Resett_switch2/1
  Relational Operator/1 -> Resett_switch1/2
  Resett_switch1/1 -> reset_old3/1
  reset_old3/1 -> Relational Operator/1, count/1, Add1/2
  speed_old_switch2/1 -> reset_old4/1
  Constant5/1 -> speed_old_switch2/3
  Dir/1 -> reset_old6/1
  IncsPerTurn/1 -> Reset_when_overflow/2, Resett_switch3/1
  Reset_when_overflow/1 -> reset_old5/1
  Constant4/1 -> Reset_when_overflow/1
  Constant2/1 -> speed_old_switch2/1
  Constant3/1 -> speed_old_switch1/3
  speed_old_switch1/1 -> Add1/1
  Add1/1 -> Resett_switch2/3
  Detec_edge/1 -> reset_old_switch1/2, speed_old_switch1/2  "1 for one cycle if edge recognized"
  reset_old1/1 -> Detec_edge/2, reset_old_switch1/3
  reset_old_switch1/1 -> reset_old1/1
  Enable_ctr/1 -> reset_old_switch1/1, Detec_edge/1
  Reset_flag/1 -> Resett_switch2/2, reset_old_switch/2
  reset_old/1 -> Reset_flag/2, reset_old_switch/3
  reset_old_switch/1 -> reset_old/1
  Reset/1 -> reset_old_switch/1, Reset_flag/1

== system gm_Encoder_Zynq_V24/IncreEncoder_V19/Counter_theta_ele ==
  note: Check if count is to small
  note: Check if count is to big
  note: Count
  note: Reset
  note: 1 for one cycle if edge recognized
  Enable_ctr : Inport
  Reset : Inport  Port=2
  IncsPerTurn : Inport  Port=3
  Dir : Inport  Port=4
  Add1 : Sum  AccumDataTypeStr=int16  OutDataTypeStr=int16
  Constant1 : Constant  Value=0  OutDataTypeStr=int16  SampleTime=-1
  Constant2 : Constant  OutDataTypeStr=int16  SampleTime=-1
  Constant3 : Constant  Value=0  OutDataTypeStr=int16  SampleTime=-1
  Constant5 : Constant  Value=-1  OutDataTypeStr=int16  SampleTime=-1
  Detec_edge : Sum  Inputs=+-  AccumDataTypeStr=int8  OutDataTypeStr=int8
  Relational Operator : RelationalOperator  Operator=>  OutDataTypeStr=boolean  RndMeth=Nearest
  Relational Operator1 : RelationalOperator  Operator=<=  OutDataTypeStr=boolean  RndMeth=Nearest
  Reset_flag : Sum  Inputs=+-  AccumDataTypeStr=uint8  OutDataTypeStr=uint8
  Resett_switch1 : Switch  Criteria=u2 ~= 0  OutDataTypeStr=int16
  Resett_switch2 : Switch  Criteria=u2 ~= 0  OutDataTypeStr=int16
  Resett_switch3 : Switch  Criteria=u2 ~= 0  OutDataTypeStr=int16
  only_use_for_neg_speed : Switch  Threshold=1
  reset_old{,1..5} (6 alike) : Delay  DelayLength=1
  reset_old_switch : Switch  Criteria=u2 ~= 0
  reset_old_switch1 : Switch  Criteria=u2 ~= 0
  speed_old_switch1 : Switch  Criteria=u2 ~= 0
  speed_old_switch2 : Switch  Threshold=1
  count : Outport
  wires:
  reset_old5/1 -> only_use_for_neg_speed/2, speed_old_switch2/2
  reset_old4/1 -> speed_old_switch1/1
  only_use_for_neg_speed/1 -> Resett_switch3/2
  Relational Operator1/1 -> only_use_for_neg_speed/3
  reset_old2/1 -> Relational Operator1/1
  Resett_switch2/1 -> Resett_switch3/3
  Resett_switch3/1 -> Resett_switch1/3, reset_old2/1
  Constant1/1 -> Resett_switch1/1, Relational Operator1/2, only_use_for_neg_speed/1, Resett_switch2/1
  Relational Operator/1 -> Resett_switch1/2
  Resett_switch1/1 -> reset_old3/1
  reset_old3/1 -> Relational Operator/1, count/1, Add1/2
  speed_old_switch2/1 -> reset_old4/1
  Constant5/1 -> speed_old_switch2/3
  Dir/1 -> reset_old5/1
  IncsPerTurn/1 -> Relational Operator/2, Resett_switch3/1
  Constant2/1 -> speed_old_switch2/1
  Constant3/1 -> speed_old_switch1/3
  speed_old_switch1/1 -> Add1/1
  Add1/1 -> Resett_switch2/3
  Detec_edge/1 -> reset_old_switch1/2, speed_old_switch1/2  "1 for one cycle if edge recognized"
  reset_old1/1 -> Detec_edge/2, reset_old_switch1/3
  reset_old_switch1/1 -> reset_old1/1
  Enable_ctr/1 -> reset_old_switch1/1, Detec_edge/1
  Reset_flag/1 -> Resett_switch2/2, reset_old_switch/2
  reset_old/1 -> Reset_flag/2, reset_old_switch/3
  reset_old_switch/1 -> reset_old/1
  Reset/1 -> reset_old_switch/1, Reset_flag/1

== system gm_Encoder_Zynq_V24/IncreEncoder_V19/n_aus_theta ==
  note: Detect each edge of the encoder
  count : Inport
  T : Inport  Port=2
  ProtectThetaLimit : Inport  Port=3
  Add : Sum  Inputs=+-
  Add1 : Sum
  Constant : Constant  Value=0  OutDataTypeStr=fixdt(0,30,24)  SampleTime=-1
  Constant1 : Constant  Value=0  OutDataTypeStr=fixdt(0,30,24)  SampleTime=-1
  Constant2 : Constant  Value=0  OutDataTypeStr=fixdt(0,30,24)  SampleTime=-1
  Logical Operator : Logic  AllPortsSameDT=off  OutDataTypeStr=boolean
  ProtectOverflow_T_count : Switch  Threshold=50
  ProtectOverflow_rps : Switch  Threshold=50  OutDataTypeStr=fixdt(0,30,24)
  ProtectToUseOmegaIfThetaJump : RelationalOperator  OutDataTypeStr=boolean  RndMeth=Nearest
  T_count : Delay  DelayLength=1
  T_count_switch : Switch  Criteria=u2 ~= 0
  count_old : Delay  DelayLength=1
  count_old_switch : Switch  Criteria=u2 ~= 0
  speed_old : Delay  DelayLength=1
  speed_old_switch : Switch  Criteria=u2 ~= 0
  rps : Outport
  wires:
  ProtectThetaLimit/1 -> ProtectToUseOmegaIfThetaJump/2
  Logical Operator/1 -> speed_old_switch/2
  ProtectToUseOmegaIfThetaJump/1 -> Logical Operator/2
  T_count_switch/1 -> ProtectOverflow_T_count/3, ProtectOverflow_T_count/2, ProtectOverflow_rps/2
  count/1 -> count_old_switch/1, Add/1, ProtectToUseOmegaIfThetaJump/1
  Add1/1 -> T_count_switch/3, speed_old_switch/1
  T_count/1 -> Add1/2
  ProtectOverflow_T_count/1 -> T_count/1
  T/1 -> Add1/1
  speed_old/1 -> speed_old_switch/3
  speed_old_switch/1 -> speed_old/1, ProtectOverflow_rps/3
  Constant2/1 -> ProtectOverflow_rps/1
  ProtectOverflow_rps/1 -> rps/1
  Constant1/1 -> ProtectOverflow_T_count/1
  Add/1 -> T_count_switch/2, Logical Operator/1, count_old_switch/2
  Constant/1 -> T_count_switch/1
  count_old/1 -> Add/2, count_old_switch/3
  count_old_switch/1 -> count_old/1

== system gm_Encoder_Zynq_V24/IncreEncoder_V22/Average ==
  note: Maximum of the OverSampling is 6
  "OmegaIn " : Inport
  NewMeasurement : Inport  Port=2
  SamplingFactorInv : Inport  Port=3
  SamplingFactor : Inport  Port=4
  Add : Sum  Inputs=++++++  OutDataTypeStr=Inherit: Same as first input
  Ask1 : Switch  Threshold=fi(2,0,4,0)  OutDataTypeStr=fixdt(1,24,11)
  Ask2 : Switch  Threshold=fi(3,0,4,0)  OutDataTypeStr=fixdt(1,24,11)
  Ask3 : Switch  Threshold=fi(4,0,4,0)  OutDataTypeStr=fixdt(1,24,11)
  Ask4 : Switch  Threshold=fi(5,0,4,0)  OutDataTypeStr=fixdt(1,24,11)
  Ask5 : Switch  Threshold=fi(6,0,4,0)  OutDataTypeStr=fixdt(1,24,11)
  Constant1 : Constant  Value=0  OutDataTypeStr=fixdt(1,24,11)  SampleTime=-1
  NewSpeed{,1..4} (5 alike) : Switch  Criteria=u2 ~= 0  Threshold=0.5  OutDataTypeStr=fixdt(1,24,11)
  Product : Product  OutDataTypeStr=Inherit: Same as first input
  hold{,1..4} (5 alike) : Delay  DelayLength=1
  OmegaOut : Outport
  wires:
  SamplingFactor/1 -> Ask5/2, Ask4/2, Ask3/2, Ask2/2, Ask1/2
  Ask5/1 -> Add/6
  Ask4/1 -> Add/5
  Ask3/1 -> Add/4
  Ask2/1 -> Add/3
  Ask1/1 -> Add/2
  Constant1/1 -> Ask1/3, Ask2/3, Ask3/3, Ask4/3, Ask5/3
  hold4/1 -> NewSpeed4/3
  NewSpeed4/1 -> Ask5/1, hold4/1
  hold3/1 -> NewSpeed3/3, NewSpeed4/1
  NewSpeed3/1 -> Ask4/1, hold3/1
  NewMeasurement/1 -> NewSpeed/2, NewSpeed1/2, NewSpeed2/2, NewSpeed3/2, NewSpeed4/2
  NewSpeed2/1 -> Ask3/1, hold2/1
  hold2/1 -> NewSpeed2/3, NewSpeed3/1
  hold1/1 -> NewSpeed1/3, NewSpeed2/1
  NewSpeed1/1 -> Ask2/1, hold1/1
  NewSpeed/1 -> Ask1/1, hold/1
  hold/1 -> NewSpeed/3, NewSpeed1/1
  Add/1 -> Product/1
  SamplingFactorInv/1 -> Product/2
  "OmegaIn "/1 -> NewSpeed/1, Add/1
  Product/1 -> OmegaOut/1

== system gm_Encoder_Zynq_V24/IncreEncoder_V22/Check_Direction ==
  A : Inport
  B : Inport  Port=2
  Add : Sum  Inputs=+-  AccumDataTypeStr=fixdt(1,4,0)  OutDataTypeStr=fixdt(1,4,0)
  Add1 : Sum  Inputs=+-  AccumDataTypeStr=fixdt(1,4,0)  OutDataTypeStr=fixdt(1,4,0)
  Add2 : Sum  AccumDataTypeStr=fixdt(1,4,0)  OutDataTypeStr=fixdt(1,4,0)
  Change : Sum  AccumDataTypeStr=fixdt(1,4,0)  OutDataTypeStr=fixdt(1,4,0)
  Change1 : Delay  DelayLength=1
  Save_Direction : Switch  Criteria=u2 ~= 0  Threshold=0.1  OutDataTypeStr=Inherit: Inherit via back propagation
  T_count_switch : Switch  Threshold=1  OutDataTypeStr=Inherit: Inherit via back propagation
  TrnLeft : Sum  Inputs=+-  AccumDataTypeStr=fixdt(1,4,0)  OutDataTypeStr=fixdt(1,4,0)
  TrnRight : Sum  Inputs=+-  AccumDataTypeStr=fixdt(1,4,0)  OutDataTypeStr=fixdt(1,4,0)
  TurnLeft : Constant  Value=-1  OutDataTypeStr=fixdt(1,4,0)  SampleTime=-1
  TurnRight : Constant  OutDataTypeStr=fixdt(1,4,0)  SampleTime=-1
  count_old : Delay  DelayLength=1
  count_old1 : Delay  DelayLength=1
  count_old2 : Delay  DelayLength=1
  count_old_switch : Switch  Criteria=u2 ~= 0  OutDataTypeStr=Inherit: Inherit via back propagation
  count_old_switch1 : Switch  Criteria=u2 ~= 0  OutDataTypeStr=Inherit: Inherit via back propagation
  new_value : Delay  DelayLength=1
  nothing : Constant  Value=0  OutDataTypeStr=fixdt(1,4,0)  SampleTime=-1
  nothing1 : Constant  Value=0  OutDataTypeStr=fixdt(1,4,0)  SampleTime=-1
  speed_old_switch : Switch  Threshold=1  OutDataTypeStr=Inherit: Inherit via back propagation
  Dir : Outport
  wires:
  count_old2/1 -> Dir/1, Save_Direction/3
  Change1/1 -> Save_Direction/2
  Change/1 -> Change1/1
  Add2/1 -> new_value/1
  speed_old_switch/1 -> Add2/2, Change/2
  nothing1/1 -> T_count_switch/3
  nothing/1 -> speed_old_switch/3
  TurnLeft/1 -> speed_old_switch/1
  TrnLeft/1 -> speed_old_switch/2
  new_value/1 -> Save_Direction/1
  TrnRight/1 -> T_count_switch/2
  Add1/1 -> count_old_switch1/2, TrnLeft/1
  count_old1/1 -> Add1/2, count_old_switch1/3
  count_old_switch1/1 -> count_old1/1
  B/1 -> count_old_switch1/1, Add1/1, TrnRight/2
  Save_Direction/1 -> count_old2/1
  T_count_switch/1 -> Add2/1, Change/1
  Add/1 -> count_old_switch/2, TrnRight/1
  TurnRight/1 -> T_count_switch/1
  count_old/1 -> Add/2, count_old_switch/3
  count_old_switch/1 -> count_old/1
  A/1 -> count_old_switch/1, Add/1, TrnLeft/2

== system gm_Encoder_Zynq_V24/IncreEncoder_V22/Counter ==
  note: Reset
  note: 1 for one cycle if edge recognized
  Enable_ctr : Inport
  I_line : Inport  Port=2
  Detec_edge : Sum  Inputs=+-  AccumDataTypeStr=int8  OutDataTypeStr=int8
  Reset_flag : Sum  Inputs=+-  AccumDataTypeStr=uint8  OutDataTypeStr=uint8
  reset_old : Delay  DelayLength=1
  reset_old1 : Delay  DelayLength=1
  reset_old_switch : Switch  Criteria=u2 ~= 0
  reset_old_switch1 : Switch  Criteria=u2 ~= 0
  Edge : Outport
  Reset : Outport  Port=2
  wires:
  Detec_edge/1 -> Edge/1, reset_old_switch1/2  "1 for one cycle if edge recognized"
  reset_old1/1 -> Detec_edge/2, reset_old_switch1/3
  reset_old_switch1/1 -> reset_old1/1
  Enable_ctr/1 -> reset_old_switch1/1, Detec_edge/1
  Reset_flag/1 -> reset_old_switch/2, Reset/1
  reset_old/1 -> Reset_flag/2, reset_old_switch/3
  reset_old_switch/1 -> reset_old/1
  I_line/1 -> reset_old_switch/1, Reset_flag/1

== system gm_Encoder_Zynq_V24/IncreEncoder_V22/Counter_theta ==
  note: Check if count is to small
  note: Check if count is to big
  note: Count
  Edge : Inport
  Reset : Inport  Port=2
  IncsPerTurn : Inport  Port=3
  Dir : Inport  Port=4
  Add1 : Sum  AccumDataTypeStr=int16  OutDataTypeStr=int16
  Constant1 : Constant  Value=0  OutDataTypeStr=int16  SampleTime=-1
  Constant2 : Constant  OutDataTypeStr=int16  SampleTime=-1
  Constant3 : Constant  Value=0  OutDataTypeStr=int16  SampleTime=-1
  Constant4 : Constant  Value=10  OutDataTypeStr=int16  SampleTime=-1
  Constant5 : Constant  Value=-1  OutDataTypeStr=int16  SampleTime=-1
  Relational Operator : RelationalOperator  Operator=>  OutDataTypeStr=boolean  RndMeth=Nearest
  Relational Operator1 : RelationalOperator  Operator=<=  OutDataTypeStr=boolean  RndMeth=Nearest
  Reset_when_overflow : Sum  OutDataTypeStr=int16
  Resett_switch1 : Switch  Criteria=u2 ~= 0  OutDataTypeStr=int16
  Resett_switch2 : Switch  Criteria=u2 ~= 0  OutDataTypeStr=int16
  Resett_switch3 : Switch  Criteria=u2 ~= 0  OutDataTypeStr=int16
  only_use_for_neg_speed : Switch  Threshold=1
  reset_old{2..6} (5 alike) : Delay  DelayLength=1
  speed_old_switch1 : Switch  Criteria=u2 ~= 0
  speed_old_switch2 : Switch  Threshold=1
  count : Outport
  wires:
  reset_old6/1 -> speed_old_switch2/2, only_use_for_neg_speed/2
  reset_old5/1 -> Relational Operator/2
  reset_old4/1 -> speed_old_switch1/1
  only_use_for_neg_speed/1 -> Resett_switch3/2
  Relational Operator1/1 -> only_use_for_neg_speed/3
  reset_old2/1 -> Relational Operator1/1
  Resett_switch2/1 -> Resett_switch3/3
  Resett_switch3/1 -> Resett_switch1/3, reset_old2/1
  Constant1/1 -> Relational Operator1/2, only_use_for_neg_speed/1, Resett_switch1/1, Resett_switch2/1
  Relational Operator/1 -> Resett_switch1/2
  Resett_switch1/1 -> reset_old3/1
  reset_old3/1 -> Relational Operator/1, count/1, Add1/2
  speed_old_switch2/1 -> reset_old4/1
  Constant5/1 -> speed_old_switch2/3
  Dir/1 -> reset_old6/1
  IncsPerTurn/1 -> Reset_when_overflow/2, Resett_switch3/1
  Reset_when_overflow/1 -> reset_old5/1
  Constant4/1 -> Reset_when_overflow/1
  Constant2/1 -> speed_old_switch2/1
  Constant3/1 -> speed_old_switch1/3
  speed_old_switch1/1 -> Add1/1
  Add1/1 -> Resett_switch2/3
  Edge/1 -> speed_old_switch1/2  "1 for one cycle if edge recognized"
  Reset/1 -> Resett_switch2/2

== system gm_Encoder_Zynq_V24/IncreEncoder_V22/Counter_theta_ele ==
  note: Check if count is to small
  note: Check if count is to big
  note: Count
  Edge : Inport
  Reset : Inport  Port=2
  IncsPerTurn : Inport  Port=3
  Dir : Inport  Port=4
  Add1 : Sum  AccumDataTypeStr=int16  OutDataTypeStr=int16
  Constant1 : Constant  Value=0  OutDataTypeStr=int16  SampleTime=-1
  Constant2 : Constant  OutDataTypeStr=int16  SampleTime=-1
  Constant3 : Constant  Value=0  OutDataTypeStr=int16  SampleTime=-1
  Constant5 : Constant  Value=-1  OutDataTypeStr=int16  SampleTime=-1
  Relational Operator : RelationalOperator  Operator=>  OutDataTypeStr=boolean  RndMeth=Nearest
  Relational Operator1 : RelationalOperator  Operator=<=  OutDataTypeStr=boolean  RndMeth=Nearest
  Resett_switch1 : Switch  Criteria=u2 ~= 0  OutDataTypeStr=int16
  Resett_switch2 : Switch  Criteria=u2 ~= 0  OutDataTypeStr=int16
  Resett_switch3 : Switch  Criteria=u2 ~= 0  OutDataTypeStr=int16
  only_use_for_neg_speed : Switch  Threshold=1
  reset_old{2..5} (4 alike) : Delay  DelayLength=1
  speed_old_switch1 : Switch  Criteria=u2 ~= 0
  speed_old_switch2 : Switch  Threshold=1
  count : Outport
  wires:
  reset_old5/1 -> only_use_for_neg_speed/2, speed_old_switch2/2
  reset_old4/1 -> speed_old_switch1/1
  only_use_for_neg_speed/1 -> Resett_switch3/2
  Relational Operator1/1 -> only_use_for_neg_speed/3
  reset_old2/1 -> Relational Operator1/1
  Resett_switch2/1 -> Resett_switch3/3
  Resett_switch3/1 -> Resett_switch1/3, reset_old2/1
  Constant1/1 -> Resett_switch1/1, Relational Operator1/2, only_use_for_neg_speed/1, Resett_switch2/1
  Relational Operator/1 -> Resett_switch1/2
  Resett_switch1/1 -> reset_old3/1
  reset_old3/1 -> Relational Operator/1, count/1, Add1/2
  speed_old_switch2/1 -> reset_old4/1
  Constant5/1 -> speed_old_switch2/3
  Dir/1 -> reset_old5/1
  IncsPerTurn/1 -> Resett_switch3/1, Relational Operator/2
  Constant2/1 -> speed_old_switch2/1
  Constant3/1 -> speed_old_switch1/3
  speed_old_switch1/1 -> Add1/1
  Add1/1 -> Resett_switch2/3
  Edge/1 -> speed_old_switch1/2  "1 for one cycle if edge recognized"
  Reset/1 -> Resett_switch2/2

== system gm_Encoder_Zynq_V24/IncreEncoder_V22/omega_by_count_lines ==
  note: Count
  note: Check if count is to big in order to safe for value overflow
  note: Set new counter value
  Edge : Inport
  Reset1 : Inport  Port=2
  IncsPerTurn : Inport  Port=3
  Add1 : Sum  AccumDataTypeStr=int16  OutDataTypeStr=int16
  Constant1 : Constant  Value=0  OutDataTypeStr=int16  SampleTime=-1
  Constant2 : Constant  OutDataTypeStr=int16  SampleTime=-1
  Constant3 : Constant  Value=0  OutDataTypeStr=int16  SampleTime=-1
  Constant4 : Constant  Value=10  OutDataTypeStr=int16  SampleTime=-1
  Relational Operator : RelationalOperator  Operator=>  OutDataTypeStr=boolean  RndMeth=Nearest
  Reset_when_overflow : Sum  OutDataTypeStr=int16
  Resett_switch1 : Switch  Criteria=u2 ~= 0  OutDataTypeStr=int16
  Resett_switch2 : Switch  Criteria=u2 ~= 0  OutDataTypeStr=int16
  reset_old{1,3..5} (4 alike) : Delay  DelayLength=1
  reset_old_switch1 : Switch  Criteria=u2 ~= 0
  speed_old_switch1 : Switch  Criteria=u2 ~= 0
  count : Outport
  wires:
  reset_old_switch1/1 -> count/1, reset_old1/1
  Reset1/1 -> Resett_switch2/2, reset_old_switch1/2  "Use new value"
  reset_old1/1 -> reset_old_switch1/3
  reset_old3/1 -> Relational Operator/1, Add1/2, reset_old_switch1/1
  Resett_switch1/1 -> reset_old3/1
  Constant4/1 -> Reset_when_overflow/1
  Constant2/1 -> reset_old4/1
  Add1/1 -> Resett_switch2/3
  IncsPerTurn/1 -> Reset_when_overflow/2
  Constant3/1 -> speed_old_switch1/3
  Constant1/1 -> Resett_switch1/1, Resett_switch2/1
  Edge/1 -> speed_old_switch1/2  "1 for one cycle if edge recognized"
  reset_old4/1 -> speed_old_switch1/1
  Resett_switch2/1 -> Resett_switch1/3
  reset_old5/1 -> Relational Operator/2
  speed_old_switch1/1 -> Add1/1
  Relational Operator/1 -> Resett_switch1/2
  Reset_when_overflow/1 -> reset_old5/1
